simulink library "Floor_in"  (R2018b)
settings: Solver=ode45  StartTime=0.0  StopTime=10.0  RelTol=1e-3  EnableMultiTasking=on
libraries: carnot x3
settings Model: Creator=bernd.hafner  LastModifiedBy=P41573
settings DataIOCC: LimitDataPoints=on  SaveFormat=Array  SignalLoggingSaveFormat=ModelDataLogs
settings OptimizationCC: ExpressionDepthLimit=2147483647  LifeSpan=inf
settings DebuggingCC: UnderspecifiedInitializationDetection=Classic  MergeDetectMultiDrivingBlocksExec=none  SolverPrmCheckMsg=warning  FcnCallInpInsideContextMsg=warning  StateNameClashWarn=warning  SFUnexpectedBacktrackingDiag=warning  SFNoUnconditionalDefaultTransitionDiag=warning  SFExecutionAtInitializationDiag=none
settings HardwareCC: ProdBitPerPointer=32  ProdBitPerSizeT=32  ProdBitPerPtrDiffT=32  ProdLargestAtomicFloat=None  ProdIntDivRoundTo=Undefined  ProdEndianess=Unspecified  ProdWordSize=32  ProdHWDeviceType=32-bit Generic
settings ModelReferenceCC: PropagateSignalLabelsOutOfModel=off
settings SFSimCC: SimUseLocalCustomCode=off
settings RTWCC: RTWUseLocalCustomCode=off
settings CodeAppCC: StateflowObjectComments=on
settings GRTTargetCC: TargetLangStandard=C89/C90 (ANSI)  GeneratePreprocessorConditionals=Disable all  CombineOutputUpdateFcns=off  GRTInterface=on
settings ConfigComp: CovMetricSettings=dw  CovHtmlReporting=on  CovSaveCumulativeToWorkspaceVar=on  CovSaveSingleToWorkspaceVar=on  CovExternalEMLEnable=off

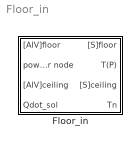
== system Floor_in ==
  Floor_in : Subsystem  mask(inner floor){wallsize=[5 5], t0=20, d=[0.015 0.38 0.02], cond=[1.4 0.79 0.7], cwall=[0.28 0.28 0.28]*3600, rho=[2000 1800 1400], misc=[0.9 0.9], dactive=-1, tau=1000*3600}
      mask prompts: wallsize "size of ceiling [m] [length width]"; t0 "initial temperature [degree centigrade]"; d "thickness of layers [m] (vector) (top to bottom)"; cond "conductivity of layers [W/(m*K)] (vector)"; cwall "capacity of nodes layers  [J/(kg*K)] (vector)"; rho "density of layers [kg/m^3]"; misc "emission_ceiling emission_floor]"; dactive "depth of the active layer(s) in m from upper surface (-1 for none)"; tau "time constant of floor [s]"
      mask help:
      | This is the model of a floor or a ceiling in a house.
      | first element of the vector = top layer (floor for room above)
      | last element of the vector = bottom layer (ceiling for room beneath)
      mask init:
      | h = wallsize(1);
      | w = wallsize(2);
      | wallsurface = h*w;
      | position = [0, 0, 0];
      | nodes = length(d);
      | 
      | emission_c = misc(1);
      | emission_f = misc(2);
      | active = 0;
      | if (dactive>=0) active=1; end
      mask Help: web(fullfile(path_carnot('help'),'Floor_in.html'),'-helpbrowser')

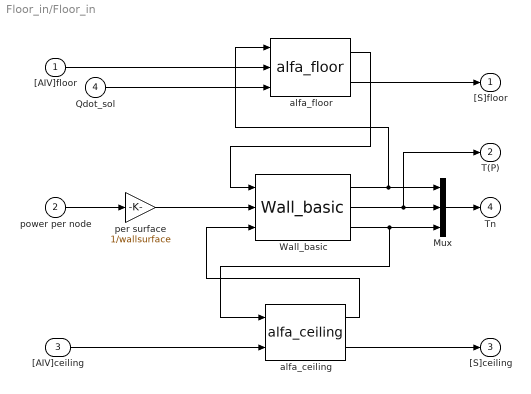
== system Floor_in/Floor_in ==
  "[AIV]floor" : Inport
  power per node : Inport  Port=2
  "[AIV]ceiling" : Inport  Port=3
  Qdot_sol : Inport  Port=4
  Mux : Mux  Inputs=3
  Wall_basic : carnot/Basic/Thermal_Models/Wall_basic  tau=tau  t0=t0  d=d  dactive=dactive  cond=cond  cwall=cwall  rho=rho
      settings: SourceProductName=Carnot
  alfa_ceiling : carnot/Basic/Heat_Transfer/alfa_ceiling  active=active  emission_c=emission_c  wallsurface=wallsurface
      settings: SourceProductName=Carnot
  alfa_floor : carnot/Basic/Heat_Transfer/alfa_floor  active=active  emission_f=emission_f  wallsurface=wallsurface
      settings: SourceProductName=Carnot
  per surface : Gain  Gain=1/wallsurface  SaturateOnIntegerOverflow=on  OutDataTypeStr=Inherit: Same as input  ParamDataTypeStr=Inherit: Same as input
  "[S]floor" : Outport
  T(P) : Outport  Port=2
  "[S]ceiling" : Outport  Port=3
  Tn : Outport  Port=4
  wires:
  Mux/1 -> Tn/1
  per surface/1 -> Wall_basic/2
  power per node/1 -> per surface/1
  Qdot_sol/1 -> alfa_floor/3
  alfa_ceiling/1 -> Wall_basic/3
  alfa_floor/1 -> Wall_basic/1
  Wall_basic/1 -> alfa_floor/1, Mux/1
  Wall_basic/3 -> alfa_ceiling/1, Mux/3
  "[AIV]floor"/1 -> alfa_floor/2
  alfa_floor/2 -> "[S]floor"/1
  alfa_ceiling/2 -> "[S]ceiling"/1
  "[AIV]ceiling"/1 -> alfa_ceiling/2
  Wall_basic/2 -> T(P)/1, Mux/2
